simulink model "untitled1"  (R2019b)
settings: Solver=VariableStepAuto  StartTime=0.0  StopTime=time  RelTol=1e-3
libraries: simulink x2
settings Model: Creator=adityaaaap  LastModifiedBy=adityaaaap

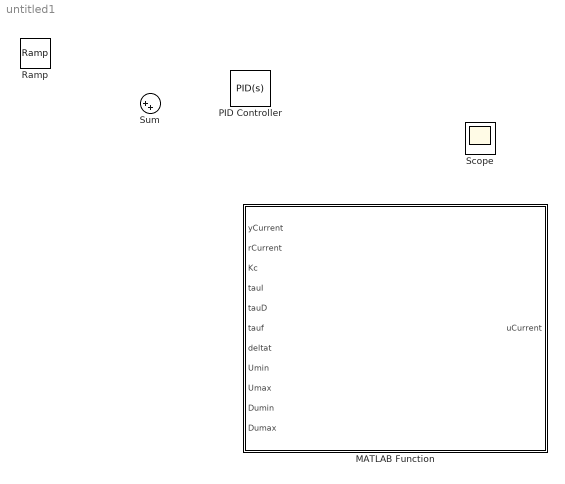
== system untitled1 ==
  MATLAB Function : MATLAB Function  TreatAsAtomicUnit=on
  PID Controller : simulink/Continuous/PID Controller  Controller=PID  Form=Parallel  TimeDomain=Continuous-time  SampleTime=-1  IntegratorMethod=Forward Euler  FilterMethod=Forward Euler  ControllerParametersSource=internal  P=1  I=1  D=0  UseFilter=on  N=100  TunerSelectOption=Transfer Function Based (PID Tuner App)  InitialConditionSource=internal  InitialConditionForIntegrator=0  InitialConditionForFilter=0  DifferentiatorICPrevScaledInput=0  ExternalReset=none  TrackingMode=off  Kt=1  LimitOutput=off  UpperSaturationLimit=inf  LowerSaturationLimit=-inf  LinearizeAsGain=on  AntiWindupMode=none  Kb=1  POutMin=[]  POutMax=[]  IOutMin=[]  IOutMax=[]  DOutMin=[]  DOutMax=[]  NOutMin=[]  NOutMax=[]  SumOutMin=[]  SumOutMax=[]  SaturationOutMin=[]  SaturationOutMax=[]  PParamMin=[]  PParamMax=[]  IParamMin=[]  IParamMax=[]  DParamMin=[]  DParamMax=[]  NParamMin=[]  NParamMax=[]  KbParamMin=[]  KbParamMax=[]  KtParamMin=[]  KtParamMax=[]  KbOutMin=[]  KbOutMax=[]  KtOutMin=[]  KtOutMax=[]  IntegratorOutMin=[]  IntegratorOutMax=[]  FilterOutMin=[]  FilterOutMax=[]  SumI1OutMin=[]  SumI1OutMax=[]  SumI2OutMin=[]  SumI2OutMax=[]  SumI3OutMin=[]  SumI3OutMax=[]  SumI4OutMin=[]  SumI4OutMax=[]  SumDOutMin=[]  SumDOutMax=[]  DifferentiatorOutMin=[]  DifferentiatorOutMax=[]  FilterDiffOutCoefMin=[]  FilterDiffOutCoefMax=[]  ReciprocalOutMin=[]  ReciprocalOutMax=[]  SumDenOutMin=[]  SumDenOutMax=[]  SumNumOutMin=[]  SumNumOutMax=[]  DivideOutMin=[]  DivideOutMax=[]  IntegratorContinuousStateAttributes=''  IntegratorStateMustResolveToSignalObject=off  IntegratorRTWStateStorageClass=Auto  FilterContinuousStateAttributes=''  FilterStateMustResolveToSignalObject=off  FilterRTWStateStorageClass=Auto  ParallelPVariant=InternalParameters  IdealPVariant=Disabled  IVariant=InternalParameters  DVariant=InternalParameters  IntegratorVariant=Continuous  SatVariant=Disabled  AWVariant=Passthrough  PCopyVariant=Disabled  TRVariant=Disabled  FdbkBlocksVariant=Forward  IdealPFdbkVariant=Disabled  SatFdbkVariant=Disabled  DerivativeFilterVariant=ContFilter  NVariant=InternalParameters  NCopyVariant=Disabled  FilterICVariant=InternalICsFilter  IntegratorICVariant=InternalICs  ExternalResetVariant=Disabled  TRSumVariant=Passthrough  SumFdbkVariant=Disabled  SumVariant=Sum_PID
  Ramp : simulink/Sources/Ramp  slope=1  start=0  InitialOutput=0
  Scope : Scope
  Sum : Sum  Inputs=|++

== matlab function untitled1/MATLAB Function ==
  data: yCurrent input; uCurrent output; rCurrent input; Kc input; tauI input; tauD input; tauf input; deltat input; Umin input; Umax input; Dumin input; Dumax input
function uCurrent = PIDV(yCurrent,rCurrent,Kc,tauI,tauD,tauf, deltat,Umin,Umax,Dumin,Dumax)
    persistent uPast 
    if isempty(uPast)
        uPast=0;
    end
    
    persistent yPast 
    if isempty(yPast)
        yPast=0; 
    end
    
    persistent uDPast 
    if isempty(uDPast)
        uDPast=0;
    end
    
    persistent rPast 
    if isempty(rPast)
        rPast=0;
    end
    
    uDCurrent=tauf/(tauf+deltat)*uDPast+(Kc*tauD)/(tauf+deltat)*(yCurrent-yPast);
    
    uCurrent=uPast+Kc*(rCurrent-yCurrent-rPast+yPast)+ (Kc*deltat)/tauI*(rCurrent-yCurrent)-uDCurrent+uDPast;
    
    uCurrent=uPast+Kc*(-yCurrent+yPast)+ (Kc*deltat)/tauI*(rCurrent-yCurrent)-uDCurrent+uDPast;
    Du=(uCurrent-uPast)/deltat;
    
    if (Du>Dumax)
        uCurrent=uPast+Dumax*deltat;
        Du=Dumax;
    end
    
    if (Du<Dumin) 
        uCurrent=uPast+Dumin*deltat;
        Du=Dumin; 
    end
    
    if (uCurrent>Umax) 
        uCurrent=Umax;
    end
    
    if (uCurrent<Umin) 
        uCurrent=Umin; 
    end
    
    uDPast=uDCurrent; 
    uPast=uCurrent; 
    yPast=yCurrent; 
    rPast=rCurrent;
end
